simulink model "ADMIRE"  (R2021b)
settings: Solver=ode4  StartTime=0.0  StopTime=100  FixedStep=1e-2  RelTol=1e-3
undefined symbols (not defined in the file or in its folder): admireDB, Earth, WGS84
libraries: simulink_extras x112, simulink x27, aerolibutil x4, dspsigops x4, aerolibfltsims x3, sharedtransform x2, aerolibtransform2 x2, aerolibatmos2 x1, matrix_library x1, sharedutil x1, aerolibanimutils x1, vrlib x1
(part 1 of 15)
settings Model: Creator=mehme  LastModifiedBy=mehme
settings DataIOCC: ExternalInput=getinputstruct(op(1))  InitialState=getstatestruct(op(1))  LoadExternalInput=on  LoadInitialState=on  SaveOutput=off  DSMLogging=off

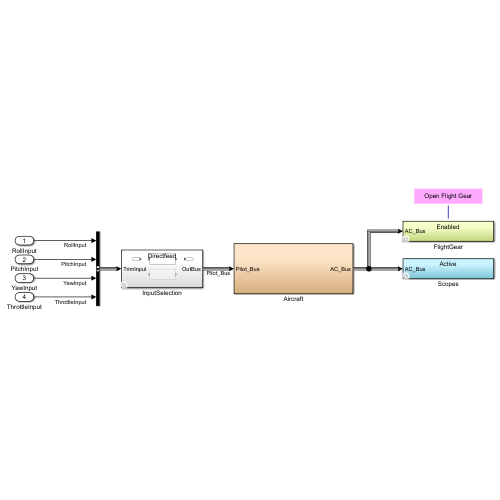
[thumbnail: Simulink's stored preview of the top-level diagram]
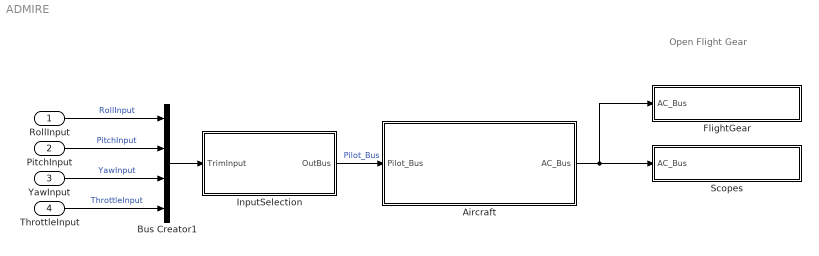
== system ADMIRE ==
  note: Open Flight Gear
  RollInput : Inport
  PitchInput : Inport  Port=2
  YawInput : Inport  Port=3
  ThrottleInput : Inport  Port=4
  Aircraft : Subsystem
  Bus Creator1 : BusCreator  Inputs=4
  FlightGear : Subsystem  Variant=on
  InputSelection : Subsystem  Variant=on  VariantControl=Choice
  Scopes : Subsystem  Variant=on  VariantControl=Choice
  wires:
  RollInput/1 -> Bus Creator1/1  "RollInput"
  YawInput/1 -> Bus Creator1/3  "YawInput"
  ThrottleInput/1 -> Bus Creator1/4  "ThrottleInput"
  Aircraft/1(AC_Bus) -> FlightGear/1(AC_Bus), Scopes/1(AC_Bus)
  PitchInput/1 -> Bus Creator1/2  "PitchInput"
  Bus Creator1/1 -> InputSelection/1(TrimInput)
  InputSelection/1(OutBus) -> Aircraft/1(Pilot_Bus)  "Pilot_Bus"

== system ADMIRE/Aircraft ==
  Pilot_Bus : Inport
  Aerodynamics : Subsystem
  AircraftPhysicalProperties : Subsystem
  Bus Creator : BusCreator  Inputs=10
  ControlSurfaces : Subsystem
  Direction Cosine Matrices : Subsystem
  Engine : Subsystem
  Environment : Subsystem
  Equtions of Motion : Subsystem
  Mass : Subsystem
  Misc : Subsystem
  AC_Bus : Outport
  wires:
  [AC_Bus] -> ControlSurfaces/1(AC_Bus), Engine/1(AC_Bus), Aerodynamics/1(AC_Bus), Equtions of Motion/1(AC_Bus), Environment/1(AC_Bus), Mass/1(Flow), Direction Cosine Matrices/1(Flow)  "AC_Bus"
  Aerodynamics/1(Aero) -> Bus Creator/5  "Aero_Bus"
  AircraftPhysicalProperties/1(ACProp) -> Bus Creator/8  "AC_Bus"
  Mass/1(Mass_Bus) -> Bus Creator/9  "Mass_Bus"
  Misc/1(Misc_Bus) -> Bus Creator/3  "Misc_Bus"
  Environment/1(Env) -> Bus Creator/7  "Env_Bus"
  Engine/1(Engine_Bus) -> Bus Creator/4  "Engine_Bus"
  Direction Cosine Matrices/1(DCM_Bus) -> Bus Creator/10  "DCM_Bus"
  Bus Creator/1 -> AC_Bus/1, [AC_Bus]
  Equtions of Motion/1(EOM_Bus) -> Bus Creator/6  "EOM_Bus"
  Pilot_Bus/1 -> Bus Creator/1  "Pilot_Bus"
  ControlSurfaces/1(CS_Bus) -> Bus Creator/2

== system ADMIRE/FlightGear ==
  AC_Bus : Inport
  Disabled : Subsystem  VariantControl=simFlag.FG == false
  Enabled : Subsystem  VariantControl=simFlag.FG == true

== system ADMIRE/InputSelection ==
  TrimInput : Inport
  Directfeed : Subsystem  VariantControl=simFlag.Input == 0
  LogitechExtremePro3D : Subsystem  VariantControl=simFlag.Input == 1
  OutBus : Outport

== system ADMIRE/Scopes ==
  AC_Bus : Inport
  Active : Subsystem  VariantControl=simFlag.Scope == 1
  Inactive : Subsystem  VariantControl=simFlag.Scope == 0

== system ADMIRE/Aircraft/Aerodynamics ==
  AC_Bus : Inport
  Bus Creator1 : BusCreator  Inputs=12
  CentripetalForceCoefficient : Subsystem
  Interface : Subsystem
  NormalForceCoefficient : Subsystem
  PitchMomentCoefficient : Subsystem
  RollMomentCoefficient : Subsystem
  Subsystem : Subsystem
  TangentialForceCoefficient : Subsystem
  YawMomentCoefficient : Subsystem
  Aero : Outport
  wires:
  AC_Bus/1 -> Subsystem/7(AC_Bus), Interface/1(AC_Bus)  "AeroIn_Bus"
  PitchMomentCoefficient/1(Cpmtot) -> Subsystem/5(cpm), Bus Creator1/5  "pitchMomentCoeff_nd"
  NormalForceCoefficient/1(Cntot) -> Subsystem/3(cn), Bus Creator1/3  "normalForceCoeff_nd"
  TangentialForceCoefficient/1(Cttot) -> Bus Creator1/1, Subsystem/1(ct)  "tangentialForceCoeff_nd"
  Bus Creator1/1 -> Aero/1  "Aero_Bus"
  Interface/1(AeroIn_Bus) -> TangentialForceCoefficient/1(AeroIn_Bus), CentripetalForceCoefficient/1(AeroIn_Bus), NormalForceCoefficient/1(AeroIn_Bus), RollMomentCoefficient/1(AeroIn_Bus), YawMomentCoefficient/1(AeroIn_Bus), PitchMomentCoefficient/1(AeroIn_Bus)  "AeroIn_Bus"
  Subsystem/1(aeroForceBodyX_N) -> Bus Creator1/7  "aeroForceBodyX_N"
  Subsystem/2(aeroForceBodyY_N) -> Bus Creator1/8  "aeroForceBodyY_N"
  Subsystem/3(aeroForceBodyZ_N) -> Bus Creator1/9  "aeroForceBodyZ_N"
  Subsystem/4(aeroMomentBodyX_N) -> Bus Creator1/10  "aeroMomentBodyX_N"
  Subsystem/5(aeroMomentBodyY_N) -> Bus Creator1/11  "aeroMomentBodyY_N"
  Subsystem/6(aeroMomentBodyZ_N) -> Bus Creator1/12  "aeroMomentBodyZ_N"
  CentripetalForceCoefficient/1(Cctot) -> Subsystem/2(cc), Bus Creator1/2  "centripetalForceCoeff_nd"
  RollMomentCoefficient/1(Crmtot) -> Subsystem/4(crm), Bus Creator1/4  "rollMomentCoeff_nd"
  YawMomentCoefficient/1(Cymtot) -> Subsystem/6(cym), Bus Creator1/6  "yawMomentCoeff_nd"

== system ADMIRE/Aircraft/AircraftPhysicalProperties ==
  Bus Creator : BusCreator  Inputs=19
  EngineOffsetY_m : Constant  Value=0
  EngineOffsetZ_m : Constant  Value=-0.15
  ReferenceAreaCanard_m2 : Constant  Value=3.20
  ReferenceAreaInboardElevon_m2 : Constant  Value=1.2
  ReferenceAreaInboardLEF_m2 : Constant  Value=0.45
  ReferenceAreaOutboardElevon_m2 : Constant  Value=1.35
  ReferenceAreaOutboardLEF_m : Constant  Value=0.45
  ReferenceAreaRudder_m2 : Constant  Value=0.80
  ReferenceArea_m2 : Constant  Value=45
  ReferenceChordCanard_m : Constant  Value=1.30
  ReferenceChordInboardElevon_m : Constant  Value=0.95
  ReferenceChordInboardLEF_m : Constant  Value=0.40
  ReferenceChordOutboardElevon_m : Constant  Value=0.68
  ReferenceChordOutboardLEF_m : Constant  Value=0.35
  ReferenceChordRudder_m : Constant  Value=0.60
  ReferenceChord_m : Constant  Value=5.2
  ReferenceLengthAirbrake_m : Constant  Value=1.10
  ReferenceSpanCanard_m : Constant  Value=2.60
  ReferenceSpan_m : Constant  Value=10
  ACProp : Outport
  wires:
  ReferenceArea_m2/1 -> Bus Creator/1  "referenceArea_m2"
  ReferenceChord_m/1 -> Bus Creator/2  "referenceChord_m"
  ReferenceSpan_m/1 -> Bus Creator/3  "referenceSpan_m"
  ReferenceAreaInboardElevon_m2/1 -> Bus Creator/4  "referenceAreaInboardElevon_m2"
  ReferenceChordInboardElevon_m/1 -> Bus Creator/5  "referenceChordInboardElevon_m"
  ReferenceAreaOutboardElevon_m2/1 -> Bus Creator/6  "referenceAreaOutboardElevon_m2"
  ReferenceChordOutboardElevon_m/1 -> Bus Creator/7  "referenceChordOutboardElevon_m"
  ReferenceAreaInboardLEF_m2/1 -> Bus Creator/8  "referenceAreaInboardLEF_m2"
  ReferenceChordInboardLEF_m/1 -> Bus Creator/9  "referenceChordInboardLEF_m"
  ReferenceAreaOutboardLEF_m/1 -> Bus Creator/10  "referenceAreaOutboardLEF_m"
  ReferenceChordOutboardLEF_m/1 -> Bus Creator/11  "referenceChordOutboardLEF_m"
  ReferenceAreaRudder_m2/1 -> Bus Creator/12  "referenceAreaRudder_m2"
  ReferenceChordRudder_m/1 -> Bus Creator/13  "referenceChordRudder_m"
  ReferenceLengthAirbrake_m/1 -> Bus Creator/14  "referenceLengthAirbrake_m"
  ReferenceAreaCanard_m2/1 -> Bus Creator/15  "referenceAreaCanard_m2"
  ReferenceChordCanard_m/1 -> Bus Creator/16  "referenceChordCanard_m"
  ReferenceSpanCanard_m/1 -> Bus Creator/17  "referenceSpanCanard_m"
  Bus Creator/1 -> ACProp/1  "AC_Bus"
  EngineOffsetY_m/1 -> Bus Creator/18  "engineOffsetY_m"
  EngineOffsetZ_m/1 -> Bus Creator/19  "engineOffsetZ_m"

== system ADMIRE/Aircraft/ControlSurfaces ==
  AC_Bus : Inport
  Actuator : Subsystem  Variant=on  VariantControl=Choice
  ControlAllocation : Subsystem
  CS_Bus : Outport
  wires:
  AC_Bus/1 -> ControlAllocation/1(AC_Bus)
  Actuator/1(actOut) -> CS_Bus/1  "CS_Bus"
  ControlAllocation/1(Cmd) -> Actuator/1(actIn)

== system ADMIRE/Aircraft/Direction Cosine Matrices ==
  Flow : Inport
  Body - Wheel : Subsystem
  Body - Wind : Subsystem
  Bus Creator : BusCreator  Inputs=6
  Earth to Body : Subsystem
  DCM_Bus : Outport
  wires:
  Flow/1 -> Body - Wheel/1(Flow), Earth to Body/1(Flow), Body - Wind/1(Flow)
  Body - Wind/1(Out1) -> Bus Creator/1  "dcmBody2Wind"
  Body - Wind/2(Out2) -> Bus Creator/2  "dcmWind2Body"
  Earth to Body/1(Out1) -> Bus Creator/3  "dcmNED2Body"
  Earth to Body/2(Out2) -> Bus Creator/4  "dcmBody2NED"
  Bus Creator/1 -> DCM_Bus/1  "DCMBuss"
  Body - Wheel/1(Out1) -> Bus Creator/5  "dcmBody2Wheel"
  Body - Wheel/2(Out2) -> Bus Creator/6  "dcmWheel2Body"

== system ADMIRE/Aircraft/Engine ==
  AC_Bus : Inport
  AB : Subsystem
  Bus Creator : BusCreator  Inputs=3
  Bus Selector : BusSelector  OutputSignals=ThrottleInput
  Ground : Ground
  Ground1 : Ground
  Interface : Subsystem
  Normal : Subsystem
  NormalAB : Subsystem
  Subsystem3 : Subsystem
  Engine_Bus : Outport
  wires:
  AC_Bus/1 -> Interface/1(AC_Bus)
  Interface/1(Out1) -> Bus Selector/1, AB/1(AC_Bus), NormalAB/1(AC_Bus), Normal/1(AC_Bus)
  Bus Selector/1 -> Subsystem3/1(tss)  "<ThrottleInput>"
  AB/1(thrustR3) -> Subsystem3/4(thrustR3)
  NormalAB/1(thrustR2) -> Subsystem3/3(thrustR2)
  Normal/1(thrustR1) -> Subsystem3/2(thrustR1)
  Bus Creator/1 -> Engine_Bus/1
  Ground/1 -> Bus Creator/2  "thrustY_N"
  Ground1/1 -> Bus Creator/3  "thrustZ_N"
  Subsystem3/1(thrust) -> Bus Creator/1  "thrustX_N"

== system ADMIRE/Aircraft/Environment ==
  AC_Bus : Inport
  Bus Creator : BusCreator  Inputs=9
  Bus Selector : BusSelector  OutputSignals=EOM_Bus.altitude_m
  Bus Selector1 : BusSelector  OutputSignals=EOM_Bus.speedWindX_mps
  Constant : Constant  Value=2
  Constant1 : Constant  Value=0.0001
  Constant2 : Constant  Value=0.5
  Constant3 : Constant  Value=0.4
  Constant4 : Constant  Value=10
  ISA Atmosphere Model : aerolibatmos2/ISA Atmosphere Model  custom=on  g=9.80665  gamma=1.4  R=287.0531  L=0.0065  h_trop=11000  h_strat=20000  rho0=1.225  P0=101325  T0=288.15  h0=0
  Power : Math  Operator=pow  SaturateOnIntegerOverflow=on
  Product : Product  Inputs=**/
  Product1 : Product
  Product2 : Product  Inputs=*/
  Product3 : Product
  Product4 : Product
  Sum : Sum  Inputs=|+-
  Sum1 : Sum  Inputs=|-+
  Env : Outport
  wires:
  AC_Bus/1 -> Bus Selector1/1, Bus Selector/1
  Bus Selector/1 -> ISA Atmosphere Model/1  "<altitude_m>"
  ISA Atmosphere Model/4 -> Product/1, Bus Creator/4  "airDensity_kgpm3"
  ISA Atmosphere Model/3 -> Bus Creator/3  "pressure_pa"
  ISA Atmosphere Model/2 -> Product2/2, Bus Creator/2  "speedOfSound_mps"
  ISA Atmosphere Model/1 -> Bus Creator/1  "temp_K"
  Bus Creator/1 -> Env/1  "Env_Bus"
  Bus Selector1/1 -> Product2/1, Power/1  "<speedWindX_mps>"
  Constant/1 -> Product/3, Power/2
  Power/1 -> Product/2
  Product/1 -> Bus Creator/5, Product1/1  "dynamicPressure_Nm2"
  Constant1/1 -> Product1/2
  Product1/1 -> Bus Creator/6  "dynamicPressure_corr"
  Constant3/1 -> Sum1/1
  Product3/1 -> Bus Creator/9  "tflow"
  Constant4/1 -> Product3/1, Product4/2
  Constant2/1 -> Sum/1
  Sum1/1 -> Product4/1
  Sum/1 -> Product3/2
  Product2/1 -> Sum/2, Sum1/2, Bus Creator/7  "mach_nd"
  Product4/1 -> Bus Creator/8  "tfhigh"

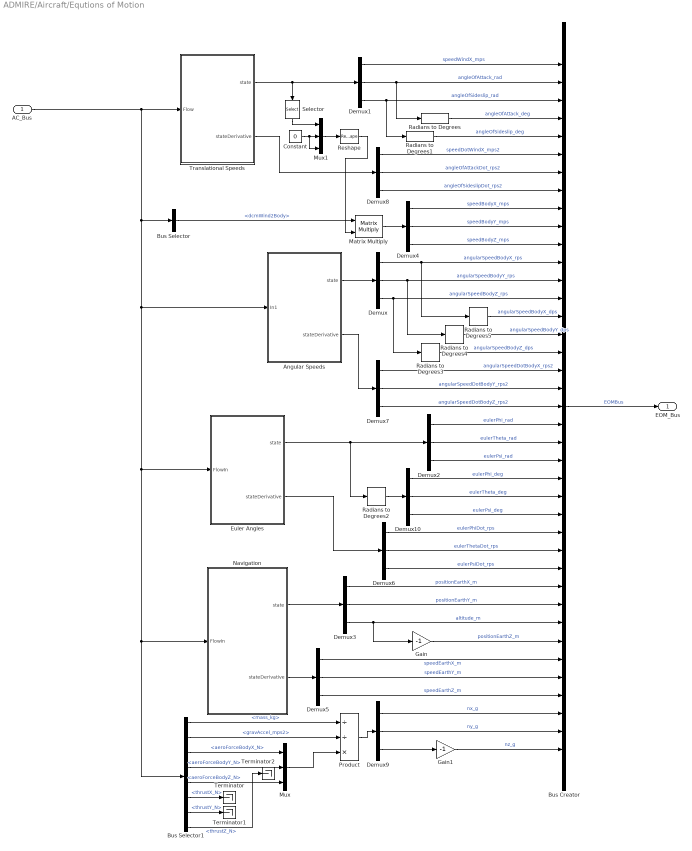
== system ADMIRE/Aircraft/Equtions of Motion ==
  AC_Bus : Inport
  Angular Speeds : Subsystem
  Bus Creator : BusCreator  Inputs=39
  Bus Selector : BusSelector  OutputSignals=DCM_Bus.dcmWind2Body
  Bus Selector1 : BusSelector  OutputSignals=Mass_Bus.mass_kg,Misc_Bus.gravAccel_mps2,Aero_Bus.aeroForceBodyX_N,Aero_Bus.aeroForceBodyY_N,Aero_Bus.aeroForceBodyZ_N,Engine_Bus.thrustX_N,Engine_Bus.thrustY_N,Engine_Bus.thrustZ_N
  Constant : Constant  Value=0
  Demux{,1..10} (11 alike) : Demux  Outputs=3
  Euler Angles : Subsystem
  Gain : Gain  Gain=-1
  Gain1 : Gain  Gain=-1
  Matrix Multiply : Product  Multiplication=Matrix(*)
  Mux : Mux  Inputs=3
  Mux1 : Mux  Inputs=3
  Navigation : Subsystem
  Product : Product  Inputs=//*
  Radians to Degrees{,1..5} (6 alike) : simulink_extras/Transformations/Radians to Degrees
  Reshape : Reshape  OutputDimensionality=Column vector (2-D)
  Selector : Selector  InputPortWidth=3  IndexOptions=Index vector (dialog)  Indices=1  OutputSizes=1
  Terminator : Terminator
  Terminator1 : Terminator
  Terminator2 : Terminator
  Translational Speeds : Subsystem
  EOM_Bus : Outport
  wires:
  AC_Bus/1 -> Translational Speeds/1(Flow), Angular Speeds/1(In1), Navigation/1(FlowIn), Bus Selector1/1, Euler Angles/1(FlowIn), Bus Selector/1
  Bus Creator/1 -> EOM_Bus/1  "EOMBus"
  Angular Speeds/1(state) -> Demux/1
  Demux/1 -> Bus Creator/12, Radians to Degrees5/1  "angularSpeedBodyX_rps"
  Demux/2 -> Bus Creator/13, Radians to Degrees4/1  "angularSpeedBodyY_rps"
  Demux/3 -> Bus Creator/14, Radians to Degrees3/1  "angularSpeedBodyZ_rps"
  Demux1/1 -> Bus Creator/1  "speedWindX_mps"
  Demux1/2 -> Radians to Degrees/1, Bus Creator/2  "angleOfAttack_rad"
  Demux1/3 -> Radians to Degrees1/1, Bus Creator/3  "angleOfSideslip_rad"
  Demux4/1 -> Bus Creator/9  "speedBodyX_mps"
  Demux4/3 -> Bus Creator/11  "speedBodyZ_mps"
  Translational Speeds/1(state) -> Demux1/1, Selector/1
  Euler Angles/1(state) -> Radians to Degrees2/1, Demux2/1
  Navigation/1(state) -> Demux3/1
  Demux3/1 -> Bus Creator/30  "positionEarthX_m"
  Demux3/2 -> Bus Creator/31  "positionEarthY_m"
  Demux3/3 -> Gain/1, Bus Creator/32  "altitude_m"
  Bus Selector/1 -> Matrix Multiply/1  "<dcmWind2Body>"
  Matrix Multiply/1 -> Demux4/1
  Demux4/2 -> Bus Creator/10  "speedBodyY_mps"
  Navigation/2(stateDerivative) -> Demux5/1
  Demux5/1 -> Bus Creator/34  "speedEarthX_m"
  Demux5/2 -> Bus Creator/35  "speedEarthY_m"
  Demux5/3 -> Bus Creator/36  "speedEarthZ_m"
  Gain/1 -> Bus Creator/33  "positionEarthZ_m"
  Demux6/2 -> Bus Creator/28  "eulerThetaDot_rps"
  Demux6/3 -> Bus Creator/29  "eulerPsiDot_rps"
  Demux6/1 -> Bus Creator/27  "eulerPhiDot_rps"
  Euler Angles/2(stateDerivative) -> Demux6/1
  Demux2/3 -> Bus Creator/23  "eulerPsi_rad"
  Demux2/2 -> Bus Creator/22  "eulerTheta_rad"
  Demux2/1 -> Bus Creator/21  "eulerPhi_rad"
  Demux7/1 -> Bus Creator/18  "angularSpeedDotBodyX_rps2"
  Demux7/3 -> Bus Creator/20  "angularSpeedDotBodyZ_rps2"
  Angular Speeds/2(stateDerivative) -> Demux7/1
  Translational Speeds/2(stateDerivative) -> Demux8/1
  Bus Selector1/5 -> Mux/3  "<aeroForceBodyZ_N>"
  Bus Selector1/4 -> Mux/2  "<aeroForceBodyY_N>"
  Bus Selector1/3 -> Mux/1  "<aeroForceBodyX_N>"
  Mux/1 -> Product/3
  Bus Selector1/2 -> Product/2  "<gravAccel_mps2>"
  Bus Selector1/1 -> Product/1  "<mass_kg>"
  Product/1 -> Demux9/1
  Demux9/1 -> Bus Creator/37  "nx_g"
  Demux9/2 -> Bus Creator/38  "ny_g"
  Gain1/1 -> Bus Creator/39  "nz_g"
  Radians to Degrees/1 -> Bus Creator/4  "angleOfAttack_deg"
  Radians to Degrees1/1 -> Bus Creator/5  "angleOfSideslip_deg"
  Radians to Degrees2/1 -> Demux10/1
  Demux10/1 -> Bus Creator/24  "eulerPhi_deg"
  Demux10/2 -> Bus Creator/25  "eulerTheta_deg"
  Demux10/3 -> Bus Creator/26  "eulerPsi_deg"
  Bus Selector1/6 -> Terminator/1  "<thrustX_N>"
  Bus Selector1/7 -> Terminator1/1  "<thrustY_N>"
  Bus Selector1/8 -> Terminator2/1  "<thrustZ_N>"
  Demux9/3 -> Gain1/1
  Demux8/3 -> Bus Creator/8  "angleOfSideslipDot_rps2"
  Demux8/2 -> Bus Creator/7  "angleOfAttackDot_rps2"
  Demux8/1 -> Bus Creator/6  "speedDotWindX_mps2"
  Demux7/2 -> Bus Creator/19  "angularSpeedDotBodyY_rps2"
  Constant/1 -> Mux1/3, Mux1/2
  Reshape/1 -> Matrix Multiply/2
  Mux1/1 -> Reshape/1
  Selector/1 -> Mux1/1
  Radians to Degrees3/1 -> Bus Creator/17  "angularSpeedBodyZ_dps"
  Radians to Degrees4/1 -> Bus Creator/16  "angularSpeedBodyY_dps"
  Radians to Degrees5/1 -> Bus Creator/15  "angularSpeedBodyX_dps"

== system ADMIRE/Aircraft/Mass ==
  Flow : Inport
  Bus Creator1 : BusCreator  Inputs=12
  Bus Selector : BusSelector  OutputSignals=DCM_Bus.dcmNED2Body
  Constant : Constant  Value=9.8065
  Constant1 : Constant  Value=0
  Constant3 : Constant  Value=0
  Demux : Demux  Outputs=3
  Inertia : Subsystem
  Matrix Multiply : Product  Multiplication=Matrix(*)
  Mux : Mux  Inputs=3
  Product : Product
  "mass " : Constant  Value=9100
  Mass_Bus : Outport
  wires:
  Bus Creator1/1 -> Mass_Bus/1  "MassBuss"
  Demux/1 -> Bus Creator1/8  "gravForceBodyX_N"
  Demux/2 -> Bus Creator1/9  "gravForceBodyY_N"
  Demux/3 -> Bus Creator1/10  "gravForceBodyZ_N"
  Constant3/1 -> Bus Creator1/11  "centerOfGravityBodyX_pct"
  "mass "/1 -> Bus Creator1/12, Product/2  "mass_kg"
  Flow/1 -> Bus Selector/1
  Constant/1 -> Product/1
  Bus Selector/1 -> Matrix Multiply/1  "<dcmNED2Body>"
  Constant1/1 -> Mux/2, Mux/1
  Product/1 -> Mux/3
  Matrix Multiply/1 -> Demux/1
  Mux/1 -> Matrix Multiply/2
  Inertia/1(InertiaTensor) -> Bus Creator1/1
  Inertia/2(inertiaIx_kgpm2) -> Bus Creator1/2
  Inertia/3(inertiaIy_kgpm2) -> Bus Creator1/3
  Inertia/4(inertiaIz_kgpm2) -> Bus Creator1/4
  Inertia/5(inertiaIxy_kgpm2) -> Bus Creator1/5
  Inertia/6(inertiaIxz_kgpm2) -> Bus Creator1/6
  Inertia/7(inertiaIyz_kgpm2) -> Bus Creator1/7

== system ADMIRE/Aircraft/Misc ==
  Bus Creator : BusCreator  Inputs=2
  Capture Air Ratio : Constant  Value=0.3
  Constant : Constant  Value=9.8065
  Misc_Bus : Outport
  wires:
  Bus Creator/1 -> Misc_Bus/1  "Misc_Bus"
  Capture Air Ratio/1 -> Bus Creator/1  "cai"
  Constant/1 -> Bus Creator/2  "gravAccel_mps2"

== system ADMIRE/FlightGear/Disabled ==
  AC_Bus : Inport
  Terminator : Terminator
  wires:
  AC_Bus/1 -> Terminator/1

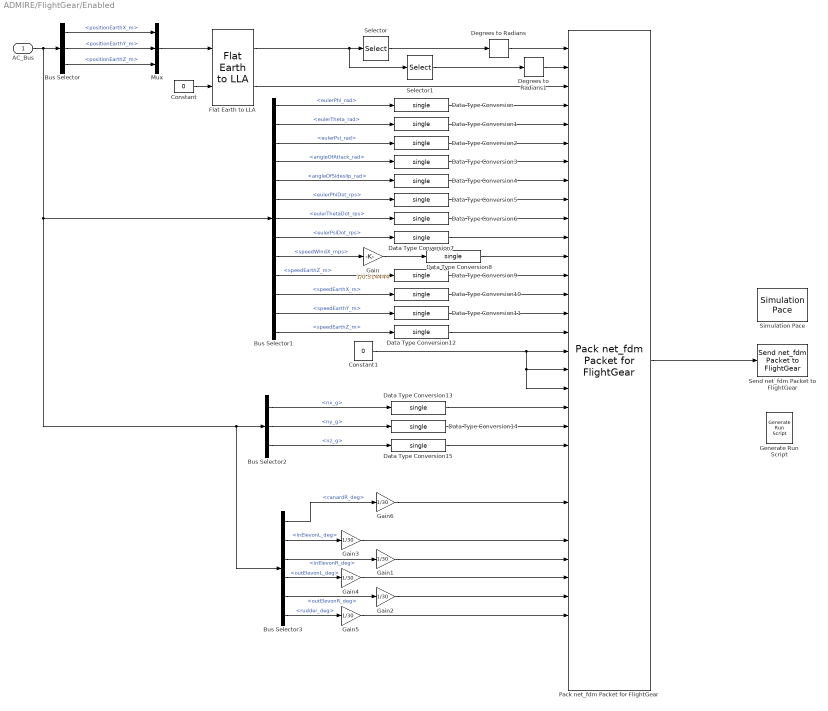
== system ADMIRE/FlightGear/Enabled ==
  AC_Bus : Inport
  Bus Selector : BusSelector  OutputSignals=EOM_Bus.positionEarthX_m,EOM_Bus.positionEarthY_m,EOM_Bus.positionEarthZ_m
  Bus Selector1 : BusSelector  OutputSignals=EOM_Bus.eulerPhi_rad,EOM_Bus.eulerTheta_rad,EOM_Bus.eulerPsi_rad,EOM_Bus.angleOfAttack_rad,EOM_Bus.angleOfSideslip_rad,EOM_Bus.eulerPhiDot_rps,EOM_Bus.eulerThetaDot_rps,EOM_Bus.eulerPsiDot_rps,EOM_Bus.speedWindX_mps,EOM_Bus.speedEarthZ_m,EOM_Bus.speedEarthX_m,EOM_Bus.speedEarthY_m,EOM_Bus.speedEarthZ_m
  Bus Selector2 : BusSelector  OutputSignals=EOM_Bus.nx_g,EOM_Bus.ny_g,EOM_Bus.nz_g
  Bus Selector3 : BusSelector  OutputSignals=CS_Bus.canardR_deg,CS_Bus.inElevonL_deg,CS_Bus.inElevonR_deg,CS_Bus.outElevonL_deg,CS_Bus.outElevonR_deg,CS_Bus.rudder_deg
  Constant : Constant  Value=0
  Constant1 : Constant  Value=0  OutDataTypeStr=single
  Data Type Conversion{,1..15} (16 alike) : DataTypeConversion  OutDataTypeStr=single
  Degrees to Radians : simulink_extras/Transformations/Degrees to Radians
  Degrees to Radians1 : simulink_extras/Transformations/Degrees to Radians
  Flat Earth to LLA : aerolibtransform2/Flat Earth to LLA  units=Metric (MKS)  ptype=Earth (WGS84)  F=1/298.257223563  R=6378137  refPosPort=off  LL0=[0 10]  psi=0
  Gain : Gain  Gain=1/0.514444
  Gain{1..6} (6 alike) : Gain  Gain=1/30  OutDataTypeStr=single
  Generate Run Script : aerolibfltsims/Generate Run Script  Architecture=Default  dataFlow=Send  GeometryModelName=gripen  AirportId=KSFO  RunwayId=10L  InitialAltitude=7224  InitialHeading=113  OffsetDistance=4.72  OffsetAzimuth=0  InstallScenery=off  DisableShaders=off  OriginAddress=127.0.0.1  DestinationPort=5502  OriginPort=5505  LocalAddress=127.0.0.1  OutputFileName=runfg.bat  FlightGearBaseDirectory=C:\Program Files\FlightGear 2024.1
  Mux : Mux  Inputs=3
  Pack net_fdm Packet for FlightGear : aerolibfltsims/Pack net_fdm Packet for FlightGear  FlightGearVersion=v2019.1  ShowPositionAttitudeInputs=on  ShowVelocityAccelerationInputs=on  ShowControlSurfacePositionInputs=on  ShowEngineFuelInputs=off  ShowLandingGearInputs=off  ShowEnvironmentInputs=off  SampleTime=-1  packetVersion=24
      settings: SourceProductBaseCode=AE
  Selector : Selector  InputPortWidth=2  IndexOptions=Index vector (dialog)  Indices=2  OutputSizes=1
  Selector1 : Selector  InputPortWidth=2  IndexOptions=Index vector (dialog)  Indices=1  OutputSizes=1
  Send net_fdm Packet to FlightGear : aerolibfltsims/Send net_fdm Packet to FlightGear  DestinationIpAddress=127.0.0.1  DestinationPort=5502  LocalIpPort=-1  varLen=off  SampleTime=-1
      settings: SourceProductBaseCode=AE
  Simulation Pace : aerolibanimutils/Simulation Pace  SimulationPace=1  SleepMode=Auto  OutputPaceError=off  SampleTime=-1
  wires:
  AC_Bus/1 -> Bus Selector3/1, Bus Selector2/1, Bus Selector1/1, Bus Selector/1
  Constant/1 -> Flat Earth to LLA/2
  Bus Selector/3 -> Mux/3  "<positionEarthZ_m>"
  Bus Selector/2 -> Mux/2  "<positionEarthY_m>"
  Bus Selector/1 -> Mux/1  "<positionEarthX_m>"
  Mux/1 -> Flat Earth to LLA/1
  Flat Earth to LLA/1 -> Selector1/1, Selector/1
  Selector/1 -> Degrees to Radians/1
  Selector1/1 -> Degrees to Radians1/1
  Flat Earth to LLA/2 -> Pack net_fdm Packet for FlightGear/3
  Bus Selector1/1 -> Data Type Conversion/1  "<eulerPhi_rad>"
  Bus Selector1/2 -> Data Type Conversion1/1  "<eulerTheta_rad>"
  Bus Selector1/3 -> Data Type Conversion2/1  "<eulerPsi_rad>"
  Bus Selector1/4 -> Data Type Conversion3/1  "<angleOfAttack_rad>"
  Bus Selector1/5 -> Data Type Conversion4/1  "<angleOfSideslip_rad>"
  Bus Selector1/6 -> Data Type Conversion5/1  "<eulerPhiDot_rps>"
  Bus Selector1/7 -> Data Type Conversion6/1  "<eulerThetaDot_rps>"
  Bus Selector1/8 -> Data Type Conversion7/1  "<eulerPsiDot_rps>"
  Bus Selector1/9 -> Gain/1  "<speedWindX_mps>"
  Gain/1 -> Data Type Conversion8/1
  Constant1/1 -> Pack net_fdm Packet for FlightGear/19, Pack net_fdm Packet for FlightGear/18, Pack net_fdm Packet for FlightGear/17
  Bus Selector1/12 -> Data Type Conversion11/1  "<speedEarthY_m>"
  Bus Selector1/11 -> Data Type Conversion10/1  "<speedEarthX_m>"
  Bus Selector1/10 -> Data Type Conversion9/1  "<speedEarthZ_m>"
  Bus Selector1/13 -> Data Type Conversion12/1  "<speedEarthZ_m>"
  Bus Selector2/1 -> Data Type Conversion13/1  "<nx_g>"
  Bus Selector2/2 -> Data Type Conversion14/1  "<ny_g>"
  Bus Selector2/3 -> Data Type Conversion15/1  "<nz_g>"
  Bus Selector3/1 -> Gain6/1  "<canardR_deg>"
  Bus Selector3/2 -> Gain3/1  "<inElevonL_deg>"
  Bus Selector3/3 -> Gain1/1  "<inElevonR_deg>"
  Bus Selector3/4 -> Gain4/1  "<outElevonL_deg>"
  Bus Selector3/5 -> Gain2/1  "<outElevonR_deg>"
  Bus Selector3/6 -> Gain5/1  "<rudder_deg>"
  Gain5/1 -> Pack net_fdm Packet for FlightGear/31
  Gain2/1 -> Pack net_fdm Packet for FlightGear/30
  Gain4/1 -> Pack net_fdm Packet for FlightGear/29
  Gain1/1 -> Pack net_fdm Packet for FlightGear/28
  Gain3/1 -> Pack net_fdm Packet for FlightGear/27
  Gain6/1 -> Pack net_fdm Packet for FlightGear/25
  Pack net_fdm Packet for FlightGear/1 -> Send net_fdm Packet to FlightGear/1
  Data Type Conversion/1 -> Pack net_fdm Packet for FlightGear/4
  Data Type Conversion1/1 -> Pack net_fdm Packet for FlightGear/5
  Data Type Conversion2/1 -> Pack net_fdm Packet for FlightGear/6
  Data Type Conversion3/1 -> Pack net_fdm Packet for FlightGear/7
  Data Type Conversion4/1 -> Pack net_fdm Packet for FlightGear/8
  Data Type Conversion5/1 -> Pack net_fdm Packet for FlightGear/9
  Data Type Conversion6/1 -> Pack net_fdm Packet for FlightGear/10
  Data Type Conversion7/1 -> Pack net_fdm Packet for FlightGear/11
  Data Type Conversion8/1 -> Pack net_fdm Packet for FlightGear/12
  Data Type Conversion9/1 -> Pack net_fdm Packet for FlightGear/13
  Data Type Conversion10/1 -> Pack net_fdm Packet for FlightGear/14
  Data Type Conversion11/1 -> Pack net_fdm Packet for FlightGear/15
  Data Type Conversion12/1 -> Pack net_fdm Packet for FlightGear/16
  Data Type Conversion13/1 -> Pack net_fdm Packet for FlightGear/20
  Data Type Conversion14/1 -> Pack net_fdm Packet for FlightGear/21
  Data Type Conversion15/1 -> Pack net_fdm Packet for FlightGear/22
  Degrees to Radians/1 -> Pack net_fdm Packet for FlightGear/1
  Degrees to Radians1/1 -> Pack net_fdm Packet for FlightGear/2

== system ADMIRE/InputSelection/Directfeed ==
  In Bus Element2 : Inport  PortName=TrimInput  Element=PitchInput
  In Bus Element3 : Inport  PortName=TrimInput  Element=YawInput
  In Bus Element4 : Inport  PortName=TrimInput  Element=ThrottleInput
  In Bus Element : Inport  PortName=TrimInput  Element=RollInput
  Bus Element Out : Outport  PortName=OutBus  Element=RollInput
  Bus Element Out1 : Outport  PortName=OutBus  Element=PitchInput
  Bus Element Out2 : Outport  PortName=OutBus  Element=YawInput
  Bus Element Out3 : Outport  PortName=OutBus  Element=ThrottleInput
  wires:
  In Bus Element/1 -> Bus Element Out/1
  In Bus Element2/1 -> Bus Element Out1/1
  In Bus Element3/1 -> Bus Element Out2/1
  In Bus Element4/1 -> Bus Element Out3/1

== system ADMIRE/InputSelection/LogitechExtremePro3D ==
  note: Ayarlanacak
  note: 1 - Roll (+ Sağ)
      | 2 - Pitch (+ Geri)
      | 3 - Yaw (+ Sağ)
      | 4 - Throttle (+ Aşağı)
  Bus Element In : Inport  PortName=TrimInput  Element=RollInput
  Bus Element In1 : Inport  PortName=TrimInput  Element=PitchInput
  Bus Element In2 : Inport  PortName=TrimInput  Element=YawInput
  Bus Element In3 : Inport  PortName=TrimInput  Element=ThrottleInput
  1-D Lookup Table : Lookup_n-D  NumberOfTableDimensions=1  BreakpointsForDimension1=[-1 -0.6 0.6 1]  Table=[+25 +10 -10 -25]  InternalRulePriority=Speed  RndMeth=Simplest  InputSameDT=on
  1-D Lookup Table1 : Lookup_n-D  NumberOfTableDimensions=1  BreakpointsForDimension1=[-1 -0.6 0.6 1]  Table=[-25 -10 10 25]  InternalRulePriority=Speed  RndMeth=Simplest  InputSameDT=on
  1-D Lookup Table2 : Lookup_n-D  NumberOfTableDimensions=1  BreakpointsForDimension1=[-1 -0.6 0.6 1]  Table=[-25 -10 10 25]  InternalRulePriority=Speed  RndMeth=Simplest  InputSameDT=on
  1-D Lookup Table3 : Lookup_n-D  NumberOfTableDimensions=1  BreakpointsForDimension1=[-1 1]  Table=[0, 1]  InternalRulePriority=Speed  RndMeth=Simplest  InputSameDT=on
  Dead Zone : DeadZone  LowerValue=-0.1  UpperValue=0.1  SaturateOnIntegerOverflow=on
  Dead Zone1 : DeadZone  LowerValue=-0.1  UpperValue=0.1  SaturateOnIntegerOverflow=on
  Dead Zone2 : DeadZone  LowerValue=-0.1  UpperValue=0.1  SaturateOnIntegerOverflow=on
  Demux : Demux
  Joystick Input : vrlib/Joystick Input  joyid=1  adjustports=on  forcefeed=off
  Subsystem : Subsystem
  Subsystem1 : Subsystem
  Subsystem2 : Subsystem
  Subsystem3 : Subsystem
  Terminator : Terminator
  Terminator1 : Terminator
  Bus Element Out : Outport  PortName=OutBus  Element=RollInput
  Bus Element Out1 : Outport  PortName=OutBus  Element=PitchInput
  Bus Element Out2 : Outport  PortName=OutBus  Element=YawInput
  Bus Element Out3 : Outport  PortName=OutBus  Element=ThrottleInput
  wires:
  Joystick Input/1 -> Demux/1
  Demux/2 -> Dead Zone1/1  "Pitch"
  Joystick Input/2 -> Terminator/1
  Demux/3 -> Dead Zone2/1  "Yaw"
  Demux/4 -> 1-D Lookup Table3/1  "Throttle"
  Joystick Input/3 -> Terminator1/1
  Demux/1 -> Dead Zone/1  "Roll"
  Bus Element In/1 -> Subsystem/2(TrimInput)
  Bus Element In1/1 -> Subsystem1/2(TrimInput)
  Bus Element In2/1 -> Subsystem2/2(TrimInput)
  Bus Element In3/1 -> Subsystem3/2(TrimInput)
  Subsystem/1(Out) -> Bus Element Out/1  "roll"
  Subsystem1/1(Out) -> Bus Element Out1/1  "pitch"
  Subsystem2/1(Out) -> Bus Element Out2/1  "yaw"
  Subsystem3/1(Out) -> Bus Element Out3/1  "throttle"
  Dead Zone/1 -> 1-D Lookup Table/1
  Dead Zone1/1 -> 1-D Lookup Table1/1
  Dead Zone2/1 -> 1-D Lookup Table2/1
  1-D Lookup Table/1 -> Subsystem/1(JoyInput)
  1-D Lookup Table1/1 -> Subsystem1/1(JoyInput)
  1-D Lookup Table2/1 -> Subsystem2/1(JoyInput)
  1-D Lookup Table3/1 -> Subsystem3/1(JoyInput)

== system ADMIRE/Scopes/Active ==
  AC_Bus : Inport
  AircraftStates : BusSelector  OutputSignals=EOM_Bus.angleOfAttack_deg,EOM_Bus.angleOfSideslip_deg,EOM_Bus.speedWindX_mps,EOM_Bus.angularSpeedBodyX_dps,EOM_Bus.angularSpeedBodyY_dps,EOM_Bus.angularSpeedBodyZ_dps,EOM_Bus.eulerPhi_deg,EOM_Bus.eulerTheta_deg,EOM_Bus.eulerPsi_deg
  ControlSurfaces : BusSelector  OutputSignals=CS_Bus.rudder_deg,CS_Bus.lef_deg,CS_Bus.lg_bool,CS_Bus.inElevonL_deg,CS_Bus.inElevonR_deg,CS_Bus.outElevonL_deg,CS_Bus.outElevonR_deg,CS_Bus.canardL_deg,CS_Bus.canardR_deg
  PilotInputs : BusSelector  OutputSignals=Pilot_Bus.RollInput,Pilot_Bus.PitchInput,Pilot_Bus.YawInput,Pilot_Bus.ThrottleInput
  Scope : Scope  NumInputPorts=4
  Scope1 : Scope  NumInputPorts=9
  Scope2 : Scope  NumInputPorts=3
  Scope3 : Scope  NumInputPorts=3
  Scope4 : Scope  NumInputPorts=3
  wires:
  AC_Bus/1 -> AircraftStates/1, ControlSurfaces/1, PilotInputs/1
  PilotInputs/1 -> Scope/1  "<RollInput>"
  PilotInputs/2 -> Scope/2  "<PitchInput>"
  PilotInputs/3 -> Scope/3  "<YawInput>"
  PilotInputs/4 -> Scope/4  "<ThrottleInput>"
  ControlSurfaces/1 -> Scope1/1  "<rudder_deg>"
  ControlSurfaces/2 -> Scope1/2  "<lef_deg>"
  ControlSurfaces/3 -> Scope1/3  "<lg_bool>"
  ControlSurfaces/4 -> Scope1/4  "<inElevonL_deg>"
  ControlSurfaces/5 -> Scope1/5  "<inElevonR_deg>"
  ControlSurfaces/6 -> Scope1/6  "<outElevonL_deg>"
  ControlSurfaces/7 -> Scope1/7  "<outElevonR_deg>"
  ControlSurfaces/8 -> Scope1/8  "<canardL_deg>"
  ControlSurfaces/9 -> Scope1/9  "<canardR_deg>"
  AircraftStates/1 -> Scope2/1  "<angleOfAttack_deg>"
  AircraftStates/2 -> Scope2/2  "<angleOfSideslip_deg>"
  AircraftStates/3 -> Scope2/3  "<speedWindX_mps>"
  AircraftStates/4 -> Scope3/1  "<angularSpeedBodyX_dps>"
  AircraftStates/5 -> Scope3/2  "<angularSpeedBodyY_dps>"
  AircraftStates/6 -> Scope3/3  "<angularSpeedBodyZ_dps>"
  AircraftStates/7 -> Scope4/1  "<eulerPhi_deg>"
  AircraftStates/8 -> Scope4/2  "<eulerTheta_deg>"
  AircraftStates/9 -> Scope4/3  "<eulerPsi_deg>"

== system ADMIRE/Scopes/Inactive ==
  AC_Bus : Inport
  Terminator : Terminator
  wires:
  AC_Bus/1 -> Terminator/1

== system ADMIRE/Aircraft/Aerodynamics/CentripetalForceCoefficient ==
  AeroIn_Bus : Inport
  Bus Selector : BusSelector  OutputSignals=mach_nd
  MachRegion1 : Subsystem
  MachRegion2 : Subsystem
  MachRegion3 : Subsystem
  MachRegion4 : Subsystem
  Subsystem : Subsystem
  Cctot : Outport
  wires:
  Subsystem/1(Cctot) -> Cctot/1
  MachRegion3/1(cctot) -> Subsystem/4(CctotMR3)
  MachRegion2/1(cctot) -> Subsystem/3(CctotMR2)
  MachRegion4/1(cttot) -> Subsystem/5(CctotMR4)
  Bus Selector/1 -> Subsystem/1(mach_nd)  "<mach_nd>"
  AeroIn_Bus/1 -> MachRegion2/1(AeroIn_Bus), MachRegion3/1(AeroIn_Bus), MachRegion4/1(AeroIn_Bus), MachRegion1/1(AeroIn_Bus), Bus Selector/1
  MachRegion1/1(cctot) -> Subsystem/2(CctotMR1)

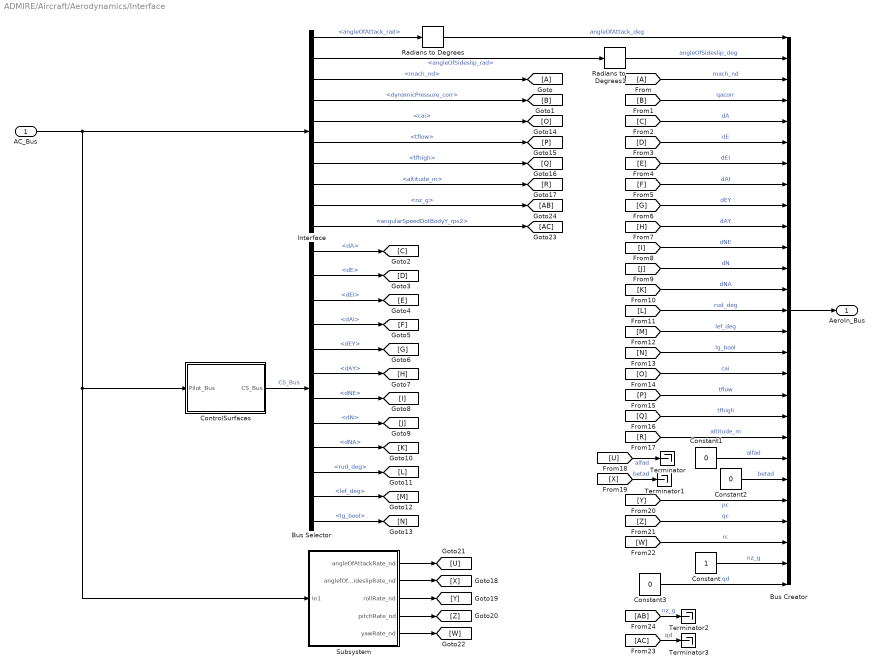
== system ADMIRE/Aircraft/Aerodynamics/Interface ==
  AC_Bus : Inport
  Bus Creator : BusCreator  Inputs=27
  Bus Selector : BusSelector  OutputSignals=dA,dE,dEI,dAI,dEY,dAY,dNE,dN,dNA,rud_deg,lef_deg,lg_bool
  Constant : Constant
  Constant1 : Constant  Value=0
  Constant2 : Constant  Value=0
  Constant3 : Constant  Value=0
  ControlSurfaces : Subsystem
  Interface : BusSelector  OutputSignals=EOM_Bus.angleOfAttack_rad,EOM_Bus.angleOfSideslip_rad,Env_Bus.mach_nd,Env_Bus.dynamicPressure_corr,Misc_Bus.cai,Env_Bus.tflow,Env_Bus.tfhigh,EOM_Bus.altitude_m,EOM_Bus.nz_g,EOM_Bus.angularSpeedDotBodyY_rps2
  Radians to Degrees : simulink_extras/Transformations/Radians to Degrees
  Radians to Degrees1 : simulink_extras/Transformations/Radians to Degrees
  Subsystem : Subsystem
  Terminator{,1..3} (4 alike) : Terminator
  AeroIn_Bus : Outport
  wires:
  AC_Bus/1 -> Subsystem/1(In1), ControlSurfaces/1(Pilot_Bus), Interface/1
  Bus Creator/1 -> AeroIn_Bus/1
  Interface/1 -> Radians to Degrees/1  "<angleOfAttack_rad>"
  Interface/2 -> Radians to Degrees1/1  "<angleOfSideslip_rad>"
  Radians to Degrees/1 -> Bus Creator/1  "angleOfAttack_deg"
  Radians to Degrees1/1 -> Bus Creator/2  "angleOfSideslip_deg"
  Interface/3 -> [A]  "<mach_nd>"
  [A] -> Bus Creator/3  "mach_nd"
  [B] -> Bus Creator/4  "qacorr"
  Interface/4 -> [B]  "<dynamicPressure_corr>"
  Interface/5 -> [O]  "<cai>"
  Interface/6 -> [P]  "<tflow>"
  Interface/7 -> [Q]  "<tfhigh>"
  Interface/8 -> [R]  "<altitude_m>"
  [C] -> Bus Creator/5  "dA"
  [D] -> Bus Creator/6  "dE"
  [E] -> Bus Creator/7  "dEI"
  [N] -> Bus Creator/16  "lg_bool"
  [F] -> Bus Creator/8  "dAI"
  [R] -> Bus Creator/20  "altitude_m"
  [O] -> Bus Creator/17  "cai"
  Constant1/1 -> Bus Creator/21  "alfad"
  Constant2/1 -> Bus Creator/22  "betad"
  [G] -> Bus Creator/9  "dEY"
  [H] -> Bus Creator/10  "dAY"
  [K] -> Bus Creator/13  "dNA"
  [L] -> Bus Creator/14  "rud_deg"
  [I] -> Bus Creator/11  "dNE"
  [J] -> Bus Creator/12  "dN"
  [M] -> Bus Creator/15  "lef_deg"
  [W] -> Bus Creator/25  "rc"
  [Q] -> Bus Creator/19  "tfhigh"
  [P] -> Bus Creator/18  "tflow"
  [Y] -> Bus Creator/23  "pc"
  [Z] -> Bus Creator/24  "qc"
  Constant/1 -> Bus Creator/26  "nz_g"
  Interface/9 -> [AB]  "<nz_g>"
  Interface/10 -> [AC]  "<angularSpeedDotBodyY_rps2>"
  Constant3/1 -> Bus Creator/27  "qd"
  Subsystem/2(anglefOfSideslipRate_nd) -> [X]
  Subsystem/1(angleOfAttackRate_nd) -> [U]
  Subsystem/3(rollRate_nd) -> [Y]
  Subsystem/4(pitchRate_nd) -> [Z]
  Subsystem/5(yawRate_nd) -> [W]
  [U] -> Terminator/1  "alfad"
  [X] -> Terminator1/1  "betad"
  [AB] -> Terminator2/1  "nz_g"
  [AC] -> Terminator3/1  "qd"
  ControlSurfaces/1(CS_Bus) -> Bus Selector/1  "CS_Bus"
  Bus Selector/1 -> [C]  "<dA>"
  Bus Selector/2 -> [D]  "<dE>"
  Bus Selector/3 -> [E]  "<dEI>"
  Bus Selector/4 -> [F]  "<dAI>"
  Bus Selector/5 -> [G]  "<dEY>"
  Bus Selector/6 -> [H]  "<dAY>"
  Bus Selector/7 -> [I]  "<dNE>"
  Bus Selector/8 -> [J]  "<dN>"
  Bus Selector/9 -> [K]  "<dNA>"
  Bus Selector/10 -> [L]  "<rud_deg>"
  Bus Selector/11 -> [M]  "<lef_deg>"
  Bus Selector/12 -> [N]  "<lg_bool>"

== system ADMIRE/Aircraft/Aerodynamics/NormalForceCoefficient ==
  AeroIn_Bus : Inport
  Bus Selector : BusSelector  OutputSignals=mach_nd
  MachRegion1 : Subsystem
  MachRegion2 : Subsystem
  MachRegion3 : Subsystem
  Subsystem : Subsystem
  Cntot : Outport
  wires:
  Subsystem/1(Cntot) -> Cntot/1
  Bus Selector/1 -> Subsystem/1(mach_nd)  "<mach_nd>"
  MachRegion2/1(Cntot) -> Subsystem/3(CntotMR2)
  AeroIn_Bus/1 -> MachRegion2/1(Misc_Bus), MachRegion3/1(Misc_Bus), MachRegion1/1(Misc_Bus), Bus Selector/1
  MachRegion3/1(Cntot) -> Subsystem/4(CntotMR3)
  MachRegion1/1(Cntot) -> Subsystem/2(CntotMR1)

== system ADMIRE/Aircraft/Aerodynamics/PitchMomentCoefficient ==
  AeroIn_Bus : Inport
  Bus Selector : BusSelector  OutputSignals=mach_nd
  MachRegion1 : Subsystem
  MachRegion2 : Subsystem
  MachRegion3 : Subsystem
  Subsystem : Subsystem
  Cpmtot : Outport
  wires:
  Subsystem/1(Cpmtot) -> Cpmtot/1
  MachRegion1/1(Cpmtot) -> Subsystem/2(CpmtotMR1)
  MachRegion2/1(Cpmtot) -> Subsystem/3(CpmtotMR2)
  MachRegion3/1(Cpmtot) -> Subsystem/4(CpmtotMR3)
  AeroIn_Bus/1 -> MachRegion2/1(Misc_Bus), MachRegion3/1(Misc_Bus), MachRegion1/1(Misc_Bus), Bus Selector/1
  Bus Selector/1 -> Subsystem/1(mach_nd)  "<mach_nd>"

== system ADMIRE/Aircraft/Aerodynamics/RollMomentCoefficient ==
  AeroIn_Bus : Inport
  Bus Selector : BusSelector  OutputSignals=mach_nd
  MachRegion1 : Subsystem
  MachRegion2 : Subsystem
  MachRegion3 : Subsystem
  MachRegion4 : Subsystem
  Subsystem : Subsystem
  Crmtot : Outport
  wires:
  Subsystem/1(Crmtot) -> Crmtot/1
  MachRegion4/1(crmtot) -> Subsystem/5(CrmtotMR4)
  MachRegion3/1(crmtot) -> Subsystem/4(CrmtotMR3)
  MachRegion2/1(crmtot) -> Subsystem/3(CrmtotMR2)
  MachRegion1/1(crmtot) -> Subsystem/2(CrmtotMR1)
  Bus Selector/1 -> Subsystem/1(mach_nd)  "<mach_nd>"
  AeroIn_Bus/1 -> MachRegion1/1(AeroIn_Bus), Bus Selector/1, MachRegion2/1(AeroIn_Bus), MachRegion3/1(AeroIn_Bus), MachRegion4/1(AeroIn_Bus)

== system ADMIRE/Aircraft/Aerodynamics/Subsystem ==
  ct : Inport
  cc : Inport  Port=2
  cn : Inport  Port=3
  crm : Inport  Port=4
  cpm : Inport  Port=5
  cym : Inport  Port=6
  AC_Bus : Inport  Port=7
  Bus Selector : BusSelector  OutputSignals=AC_Bus.referenceArea_m2,Env_Bus.dynamicPressure_Nm2
  Bus Selector1 : BusSelector  OutputSignals=AC_Bus.referenceChord_m,AC_Bus.referenceSpan_m
  Bus Selector2 : BusSelector  OutputSignals=EOM_Bus.angleOfAttack_rad
  Constant : Constant  Value=-1
  Product{,7..10} (5 alike) : Product
  Product{1..6} (6 alike) : Product  Inputs=3
  Sin : Trigonometry
  Sin1 : Trigonometry  Operator=cos
  Sum : Sum  Inputs=++|
  Sum1 : Sum  Inputs=|+-
  cd : Display
  cl : Display
  cnn : Display
  ctt : Display
  aeroForceBodyX_N : Outport
  aeroForceBodyY_N : Outport  Port=2
  aeroForceBodyZ_N : Outport  Port=3
  aeroMomentBodyX_N : Outport  Port=4
  aeroMomentBodyY_N : Outport  Port=5
  aeroMomentBodyZ_N : Outport  Port=6
  wires:
  AC_Bus/1 -> Bus Selector2/1, Bus Selector1/1, Bus Selector/1
  Bus Selector/1 -> Product/1  "<referenceArea_m2>"
  Bus Selector/2 -> Product/2  "<dynamicPressure_Nm2>"
  Product/1 -> Product6/2, Product5/2, Product4/2, Product3/2, Product2/2, Product1/2
  Constant/1 -> Product3/3, Product2/3, Product1/3
  Product3/1 -> aeroForceBodyZ_N/1
  Product2/1 -> aeroForceBodyY_N/1
  Bus Selector1/1 -> Product5/3  "<referenceChord_m>"
  Bus Selector1/2 -> Product4/3, Product6/3  "<referenceSpan_m>"
  Product6/1 -> aeroMomentBodyZ_N/1
  Product5/1 -> aeroMomentBodyY_N/1
  Product4/1 -> aeroMomentBodyX_N/1
  Product1/1 -> aeroForceBodyX_N/1
  cym/1 -> Product6/1
  cpm/1 -> Product5/1
  crm/1 -> Product4/1
  ct/1 -> Product10/2, Product8/1, ctt/1, Product1/1
  cc/1 -> Product2/1
  cn/1 -> cnn/1, Product9/2, Product7/2, Product3/1
  Bus Selector2/1 -> Sin1/1, Sin/1  "<angleOfAttack_rad>"
  Sin/1 -> Product10/1, Product7/1
  Product7/1 -> Sum/2
  Sin1/1 -> Product9/1, Product8/2
  Product8/1 -> Sum/1
  Sum/1 -> cd/1
  Product9/1 -> Sum1/1
  Product10/1 -> Sum1/2
  Sum1/1 -> cl/1

== system ADMIRE/Aircraft/Aerodynamics/TangentialForceCoefficient ==
  AeroIn_Bus : Inport
  Bus Selector : BusSelector  OutputSignals=mach_nd
  MachRegion1 : Subsystem
  MachRegion2 : Subsystem
  MachRegion3 : Subsystem
  Subsystem : Subsystem
  Cttot : Outport
  wires:
  Subsystem/1(Out1) -> Cttot/1
  MachRegion3/1(cttotMR3) -> Subsystem/4(cttotMR3)
  MachRegion2/1(cttotMR2) -> Subsystem/3(cttotMR2)
  MachRegion1/1(cttotMR1) -> Subsystem/2(cttotMR1)
  Bus Selector/1 -> Subsystem/1(mach_nd)  "<mach_nd>"
  AeroIn_Bus/1 -> MachRegion1/1(AeroIn_Bus), MachRegion2/1(AeroIn_Bus), MachRegion3/1(AeroIn_Bus), Bus Selector/1  "AeroIn_Bus"

== system ADMIRE/Aircraft/Aerodynamics/YawMomentCoefficient ==
  AeroIn_Bus : Inport
  Bus Selector : BusSelector  OutputSignals=mach_nd
  MachRegion1 : Subsystem
  MachRegion2 : Subsystem
  MachRegion3 : Subsystem
  MachRegion4 : Subsystem
  Subsystem : Subsystem
  Cymtot : Outport
  wires:
  Subsystem/1(Cymtot) -> Cymtot/1
  Bus Selector/1 -> Subsystem/1(mach_nd)  "<mach_nd>"
  MachRegion1/1(Cymtot) -> Subsystem/2(CymtotMR1)
  MachRegion3/1(Cymtot) -> Subsystem/4(CymtotMR3)
  AeroIn_Bus/1 -> MachRegion1/1(AeroIn_Bus), Bus Selector/1, MachRegion2/1(AeroIn_Bus), MachRegion3/1(AeroIn_Bus), MachRegion4/1(AeroIn_Bus)
  MachRegion4/1(Cymtot) -> Subsystem/5(CymtotMR4)
  MachRegion2/1(Cymtot) -> Subsystem/3(CymtotMR2)

== system ADMIRE/Aircraft/ControlSurfaces/Actuator ==
  actIn : Inport
  Directfeed : Subsystem  VariantControl=simFlag.Actuator == 0
  FirstOrder : Subsystem  VariantControl=simFlag.Actuator == 1
  actOut : Outport

== system ADMIRE/Aircraft/ControlSurfaces/ControlAllocation ==
  AC_Bus : Inport
  Bus Creator : BusCreator  Inputs=10
  Bus Selector : BusSelector  OutputSignals=Pilot_Bus.RollInput,Pilot_Bus.PitchInput,Pilot_Bus.YawInput,Pilot_Bus.ThrottleInput
  Gain{,2..5} (5 alike) : Gain
  Gain1 : Gain  Gain=-1
  LeadingEdgeFlap_rad : Constant  Value=0
  LeftInboardElevon_rad : Constant  Value=0
  RightInboardElevon_rad : Constant  Value=0
  dlg : Constant  Value=0
  Cmd : Outport
  wires:
  AC_Bus/1 -> Bus Selector/1
  Bus Selector/1 -> Gain/1, Gain1/1  "<RollInput>"
  Gain/1 -> Bus Creator/1  "outElevonRCmd_deg"
  Gain1/1 -> Bus Creator/6  "outElevonLCmd_deg"
  Bus Selector/2 -> Gain2/1, Gain3/1  "<PitchInput>"
  Gain2/1 -> Bus Creator/2  "canardRCmd_deg"
  Gain3/1 -> Bus Creator/5  "canardLCmd_deg"
  Bus Selector/3 -> Gain4/1  "<YawInput>"
  Gain4/1 -> Bus Creator/3  "rudderCmd_deg"
  Bus Selector/4 -> Gain5/1  "<ThrottleInput>"
  Gain5/1 -> Bus Creator/4  "thrustCmd_pct"
  Bus Creator/1 -> Cmd/1
  LeftInboardElevon_rad/1 -> Bus Creator/7  "inElevonLCmd_deg"
  RightInboardElevon_rad/1 -> Bus Creator/8  "inElevonRCmd_deg"
  LeadingEdgeFlap_rad/1 -> Bus Creator/9  "lefCmd_deg"
  dlg/1 -> Bus Creator/10  "lgCmd_bool"

== system ADMIRE/Aircraft/Direction Cosine Matrices/Body - Wheel ==
  Flow : Inport
  Bus Selector : BusSelector  OutputSignals=EOM_Bus.eulerPhi_rad,EOM_Bus.eulerTheta_rad
  Constant : Constant  Value=0
  Constant1 : Constant  Value=-1
  Invert 3x3 Matrix : aerolibutil/Invert  3x3 Matrix
  Mux : Mux  Inputs=3
  Product : Product
  Product1 : Product
  Rotation Angles to Direction Cosine Matrix : sharedtransform/Rotation Angles to Direction Cosine Matrix  rotationOrder=ZXY  aMode=aMode
      settings: SourceProductBaseCode=AE,PW,DR,MT,UV,VE
  Out1 : Outport
  Out2 : Outport  Port=2
  wires:
  Flow/1 -> Bus Selector/1
  Product/1 -> Mux/2
  Mux/1 -> Rotation Angles to Direction Cosine Matrix/1
  Rotation Angles to Direction Cosine Matrix/1 -> Out1/1, Invert 3x3 Matrix/1  "dcmBody2Wheel"
  Product1/1 -> Mux/3
  Invert 3x3 Matrix/1 -> Out2/1  "dcmWheel2Body"
  Constant/1 -> Mux/1  "<eulerPsi_rad>"
  Bus Selector/2 -> Product1/2  "<eulerTheta_rad>"
  Bus Selector/1 -> Product/1  "<eulerPhi_rad>"
  Constant1/1 -> Product/2, Product1/1

== system ADMIRE/Aircraft/Direction Cosine Matrices/Body - Wind ==
  Flow : Inport
  Bus Selector : BusSelector  OutputSignals=EOM_Bus.angleOfAttack_rad,EOM_Bus.angleOfSideslip_rad
  Direction Cosine Matrix Body to Wind : aerolibtransform2/Direction Cosine Matrix Body to Wind
      settings: SourceProductBaseCode=AE
  Invert 3x3 Matrix : aerolibutil/Invert  3x3 Matrix
  Mux : Mux  Inputs=2
  Out1 : Outport
  Out2 : Outport  Port=2
  wires:
  Flow/1 -> Bus Selector/1
  Bus Selector/1 -> Mux/1  "<angleOfAttack_rad>"
  Bus Selector/2 -> Mux/2  "<angleOfSideslip_rad>"
  Mux/1 -> Direction Cosine Matrix Body to Wind/1
  Direction Cosine Matrix Body to Wind/1 -> Out1/1, Invert 3x3 Matrix/1  "dcmBody2Wind"
  Invert 3x3 Matrix/1 -> Out2/1  "dcmWind2Body"

== system ADMIRE/Aircraft/Direction Cosine Matrices/Earth to Body ==
  Flow : Inport
  Bus Selector : BusSelector  OutputSignals=EOM_Bus.eulerPsi_rad,EOM_Bus.eulerTheta_rad,EOM_Bus.eulerPhi_rad
  Invert 3x3 Matrix : aerolibutil/Invert  3x3 Matrix
  Mux : Mux  Inputs=3
  Rotation Angles to Direction Cosine Matrix : sharedtransform/Rotation Angles to Direction Cosine Matrix  rotationOrder=ZYX  aMode=aMode
      settings: SourceProductBaseCode=AE,PW,DR,MT,UV,VE
  Out1 : Outport
  Out2 : Outport  Port=2
  wires:
  Invert 3x3 Matrix/1 -> Out2/1  "dcmBody2NED"
  Rotation Angles to Direction Cosine Matrix/1 -> Invert 3x3 Matrix/1, Out1/1  "dcmNED2Body"
  Mux/1 -> Rotation Angles to Direction Cosine Matrix/1
  Bus Selector/2 -> Mux/2  "<eulerTheta_rad>"
  Bus Selector/1 -> Mux/1  "<eulerPsi_rad>"
  Flow/1 -> Bus Selector/1
  Bus Selector/3 -> Mux/3  "<eulerPhi_rad>"

== system ADMIRE/Aircraft/Engine/AB ==
  AC_Bus : Inport
  Bus Selector : BusSelector  OutputSignals=mach_nd,altitude_m,ThrottleInput
  THRUST02_M_ALT_TSS : Lookup_n-D  NumberOfTableDimensions=3  BreakpointsForDimension1=admireDB.aerodata_thrust02.thrust02.breakpoints.M  BreakpointsForDimension2=admireDB.aerodata_thrust02.thrust02.breakpoints.ALT  BreakpointsForDimension3=admireDB.aerodata_thrust02.thrust02.breakpoints.TSS  Table=admireDB.aerodata_thrust02.thrust02.newTable  InternalRulePriority=Speed  RndMeth=Simplest  InputSameDT=on
      settings: InputPortMap=u0,u1,u2
  thrustR3 : Outport
  wires:
  THRUST02_M_ALT_TSS/1 -> thrustR3/1
  Bus Selector/3 -> THRUST02_M_ALT_TSS/3  "<ThrottleInput>"
  Bus Selector/1 -> THRUST02_M_ALT_TSS/1  "<mach_nd>"
  Bus Selector/2 -> THRUST02_M_ALT_TSS/2  "<altitude_m>"
  AC_Bus/1 -> Bus Selector/1

== system ADMIRE/Aircraft/Engine/Interface ==
  AC_Bus : Inport
  Bus Creator : BusCreator  Inputs=3
  Bus Selector : BusSelector  OutputSignals=Pilot_Bus.ThrottleInput,EOM_Bus.altitude_m,Env_Bus.mach_nd
  Out1 : Outport
  wires:
  AC_Bus/1 -> Bus Selector/1
  Bus Selector/1 -> Bus Creator/1  "<ThrottleInput>"
  Bus Selector/2 -> Bus Creator/2  "<altitude_m>"
  Bus Selector/3 -> Bus Creator/3  "<mach_nd>"
  Bus Creator/1 -> Out1/1

== system ADMIRE/Aircraft/Engine/Normal ==
  AC_Bus : Inport
  Bus Selector : BusSelector  OutputSignals=mach_nd,altitude_m,ThrottleInput
  THRUST01_M_ALT_TSS : Lookup_n-D  NumberOfTableDimensions=3  BreakpointsForDimension1=admireDB.aerodata_thrust01.thrust01.breakpoints.M  BreakpointsForDimension2=admireDB.aerodata_thrust01.thrust01.breakpoints.ALT  BreakpointsForDimension3=admireDB.aerodata_thrust01.thrust01.breakpoints.TSS  Table=admireDB.aerodata_thrust01.thrust01.newTable  InternalRulePriority=Speed  RndMeth=Simplest  InputSameDT=on
      settings: InputPortMap=u0,u1,u2
  thrustR1 : Outport
  wires:
  AC_Bus/1 -> Bus Selector/1
  Bus Selector/2 -> THRUST01_M_ALT_TSS/2  "<altitude_m>"
  Bus Selector/1 -> THRUST01_M_ALT_TSS/1  "<mach_nd>"
  Bus Selector/3 -> THRUST01_M_ALT_TSS/3  "<ThrottleInput>"
  THRUST01_M_ALT_TSS/1 -> thrustR1/1

== system ADMIRE/Aircraft/Engine/NormalAB ==
  AC_Bus : Inport
  Bus Selector : BusSelector  OutputSignals=ThrottleInput,mach_nd,altitude_m
  Constant : Constant  Value=0.78
  Constant1 : Constant  Value=0.82
  Constant2 : Constant  Value=0.78
  Constant3 : Constant  Value=25
  Product : Product  Inputs=3
  Sum : Sum  Inputs=|+-
  Sum1 : Sum  Inputs=-+|
  Sum2 : Sum  Inputs=|++
  THRUST01_M_ALT_TSS : Lookup_n-D  NumberOfTableDimensions=3  BreakpointsForDimension1=admireDB.aerodata_thrust01.thrust01.breakpoints.M  BreakpointsForDimension2=admireDB.aerodata_thrust01.thrust01.breakpoints.ALT  BreakpointsForDimension3=admireDB.aerodata_thrust01.thrust01.breakpoints.TSS  Table=admireDB.aerodata_thrust01.thrust01.newTable  InternalRulePriority=Speed  RndMeth=Simplest  InputSameDT=on
      settings: InputPortMap=u0,u1,u2
  THRUST02_M_ALT_TSS : Lookup_n-D  NumberOfTableDimensions=3  BreakpointsForDimension1=admireDB.aerodata_thrust02.thrust02.breakpoints.M  BreakpointsForDimension2=admireDB.aerodata_thrust02.thrust02.breakpoints.ALT  BreakpointsForDimension3=admireDB.aerodata_thrust02.thrust02.breakpoints.TSS  Table=admireDB.aerodata_thrust02.thrust02.newTable  InternalRulePriority=Speed  RndMeth=Simplest  InputSameDT=on
      settings: InputPortMap=u0,u1,u2
  thrustR2 : Outport
  wires:
  THRUST01_M_ALT_TSS/1 -> Sum2/2, Sum/2  "Thrust_low"
  Bus Selector/2 -> THRUST01_M_ALT_TSS/1, THRUST02_M_ALT_TSS/1  "<mach_nd>"
  Bus Selector/3 -> THRUST01_M_ALT_TSS/2, THRUST02_M_ALT_TSS/2  "<altitude_m>"
  AC_Bus/1 -> Bus Selector/1
  Constant/1 -> THRUST01_M_ALT_TSS/3
  Constant1/1 -> THRUST02_M_ALT_TSS/3
  THRUST02_M_ALT_TSS/1 -> Sum/1  "Thrust_high"
  Bus Selector/1 -> Sum1/2  "<ThrottleInput>"
  Constant2/1 -> Sum1/1
  Sum1/1 -> Product/1
  Sum/1 -> Product/3
  Constant3/1 -> Product/2
  Product/1 -> Sum2/1
  Sum2/1 -> thrustR2/1

== system ADMIRE/Aircraft/Engine/Subsystem3 ==
  tss : Inport
  thrustR1 : Inport  Port=2
  thrustR2 : Inport  Port=3
  thrustR3 : Inport  Port=4
  AND : Logic  IconShape=distinctive  AllPortsSameDT=off  OutDataTypeStr=boolean
  Compare To Constant1 : simulink/Logic and Bit Operations/Compare To Constant  relop=<  const=0.78  OutDataTypeStr=boolean
  Compare To Constant2 : simulink/Logic and Bit Operations/Compare To Constant  relop=>=  const=0.78  OutDataTypeStr=boolean
  Compare To Constant3 : simulink/Logic and Bit Operations/Compare To Constant  relop=<  const=0.82  OutDataTypeStr=boolean
  Switch : Switch  Criteria=u2 ~= 0
  Switch1 : Switch  Criteria=u2 ~= 0
  thrust : Outport
  wires:
  tss/1 -> Compare To Constant2/1, Compare To Constant3/1, Compare To Constant1/1
  Compare To Constant1/1 -> Switch/2
  Compare To Constant2/1 -> AND/1
  Compare To Constant3/1 -> AND/2
  AND/1 -> Switch1/2
  thrustR1/1 -> Switch/1
  Switch1/1 -> Switch/3
  thrustR2/1 -> Switch1/1
  thrustR3/1 -> Switch1/3
  Switch/1 -> thrust/1

== system ADMIRE/Aircraft/Equtions of Motion/Angular Speeds ==
  In1 : Inport
  Bus Selector : BusSelector  OutputSignals=Mass_Bus.InertiaTensor,EOM_Bus.angularSpeedBodyX_rps,EOM_Bus.angularSpeedBodyY_rps,EOM_Bus.angularSpeedBodyZ_rps
  Cross Product : matrix_library/Cross Product
      settings: SourceProductBaseCode=SL
  Demux : Demux  Outputs=3
  Invert 3x3 Matrix : aerolibutil/Invert  3x3 Matrix
  Matrix Multiply : Product  Multiplication=Matrix(*)
  Matrix Multiply1 : Product  Multiplication=Matrix(*)
  Mux1 : Mux  Inputs=3
  Mux2 : Mux  Inputs=3
  Reshape : Reshape  OutputDimensionality=Column vector (2-D)
  Subsystem : Subsystem
  Sum : Sum  Inputs=|-+
  angularSpeedBodyX_rps : Integrator  ContinuousStateAttributes='angularSpeedBodyX_rps'
  angularSpeedBodyY_rps : Integrator  ContinuousStateAttributes='angularSpeedBodyY_rps'
  angularSpeedBodyZ_rps : Integrator  ContinuousStateAttributes='angularSpeedBodyZ_rps'
  state : Outport
  stateDerivative : Outport  Port=2
  wires:
  In1/1 -> Subsystem/1(In1), Bus Selector/1
  Bus Selector/1 -> Invert 3x3 Matrix/1, Matrix Multiply1/1  "<InertiaTensor>"
  Bus Selector/2 -> Mux1/1  "<angularSpeedBodyX_rps>"
  Bus Selector/3 -> Mux1/2  "<angularSpeedBodyY_rps>"
  Bus Selector/4 -> Mux1/3  "<angularSpeedBodyZ_rps>"
  Cross Product/1 -> Sum/1
  Invert 3x3 Matrix/1 -> Matrix Multiply/1
  Matrix Multiply/1 -> stateDerivative/1, Demux/1
  Mux1/1 -> Matrix Multiply1/2, Cross Product/1
  Matrix Multiply1/1 -> Cross Product/2
  Sum/1 -> Reshape/1
  Demux/1 -> angularSpeedBodyX_rps/1
  Demux/2 -> angularSpeedBodyY_rps/1
  Demux/3 -> angularSpeedBodyZ_rps/1
  angularSpeedBodyX_rps/1 -> Mux2/1
  angularSpeedBodyY_rps/1 -> Mux2/2
  angularSpeedBodyZ_rps/1 -> Mux2/3
  Mux2/1 -> state/1
  Subsystem/1(Out1) -> Sum/2
  Reshape/1 -> Matrix Multiply/2
